simulink library "Library_Steering"  (R2023a)
settings: Solver=VariableStepAuto  StartTime=0.0  StopTime=10.0  RelTol=1e-3
undefined symbols (not defined in the file or in its folder): SteeringLeft, SteeringRight
libraries: mbd_s32k1xx_ec_toolbox x17, simulink x8, $bdroot x3
(part 1 of 2)
settings Model: Creator=cbeal  LastModifiedBy=cbeal
settings SolverCC: AlgebraicLoopSolver=TrustRegion
settings DebuggingCC: UnconnectedInputMsg=warning  UnconnectedOutputMsg=warning  UnconnectedLineMsg=warning
settings ModelReferenceCC: EnableRefExpFcnMdlSchedulingChecks=on
settings RTWCC: DLArmComputeVersion=19.05

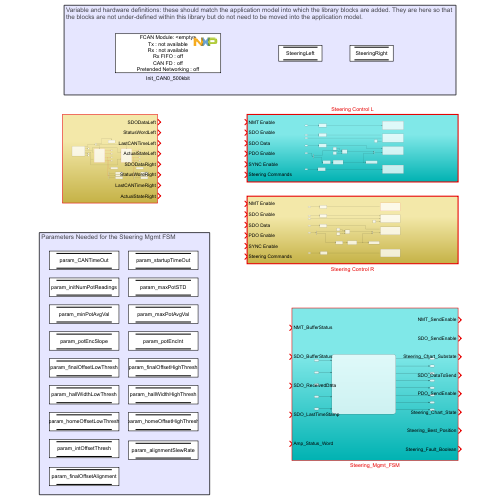
[thumbnail: Simulink's stored preview of the top-level diagram]
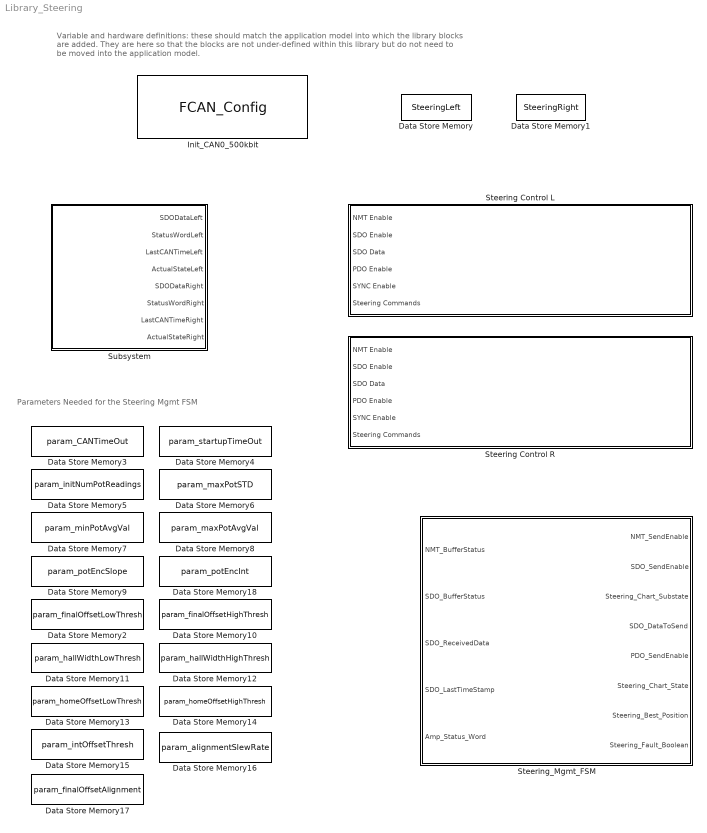
== system Library_Steering ==
  note: Parameters Needed for the Steering Mgmt FSM
  note: Variable and hardware definitions: these should match the application model into which the library blocks are added. They are here so that
      | the blocks are not under-defined within this library but do not need to be moved into the application model.
  Data Store Memory : DataStoreMemory  DataStoreName=SteeringLeft  ReadBeforeWriteMsg=warning  WriteAfterWriteMsg=warning  WriteAfterReadMsg=warning  InitialValue=zeros(15,1)  ShowAdditionalParam=off  OutDataTypeStr=uint8
  Data Store Memory1 : DataStoreMemory  DataStoreName=SteeringRight  ReadBeforeWriteMsg=warning  WriteAfterWriteMsg=warning  WriteAfterReadMsg=warning  InitialValue=zeros(15,1)  ShowAdditionalParam=off  OutDataTypeStr=uint8
  Data Store Memory10 : DataStoreMemory  DataStoreName=param_finalOffsetHighThresh  ReadBeforeWriteMsg=warning  WriteAfterWriteMsg=warning  WriteAfterReadMsg=warning  InitialValue=p1params.steering.left.finalOffsetHighThresh  ShowAdditionalParam=off  OutDataTypeStr=double
  Data Store Memory11 : DataStoreMemory  DataStoreName=param_hallWidthLowThresh  ReadBeforeWriteMsg=warning  WriteAfterWriteMsg=warning  WriteAfterReadMsg=warning  InitialValue=p1params.steering.left.hallWidthLowThresh  ShowAdditionalParam=off  OutDataTypeStr=double
  Data Store Memory12 : DataStoreMemory  DataStoreName=param_hallWidthHighThresh  ReadBeforeWriteMsg=warning  WriteAfterWriteMsg=warning  WriteAfterReadMsg=warning  InitialValue=p1params.steering.left.hallWidthHighThresh  ShowAdditionalParam=off  OutDataTypeStr=double
  Data Store Memory13 : DataStoreMemory  DataStoreName=param_homeOffsetLowThresh  ReadBeforeWriteMsg=warning  WriteAfterWriteMsg=warning  WriteAfterReadMsg=warning  InitialValue=p1params.steering.left.homeOffsetLowThresh  ShowAdditionalParam=off  OutDataTypeStr=double
  Data Store Memory14 : DataStoreMemory  DataStoreName=param_homeOffsetHighThresh  ReadBeforeWriteMsg=warning  WriteAfterWriteMsg=warning  WriteAfterReadMsg=warning  InitialValue=p1params.steering.left.homeOffsetHighThresh  ShowAdditionalParam=off  OutDataTypeStr=double
  Data Store Memory15 : DataStoreMemory  DataStoreName=param_intOffsetThresh  ReadBeforeWriteMsg=warning  WriteAfterWriteMsg=warning  WriteAfterReadMsg=warning  InitialValue=p1params.steering.left.intOffsetThresh  ShowAdditionalParam=off  OutDataTypeStr=double
  Data Store Memory16 : DataStoreMemory  DataStoreName=param_alignmentSlewRate  ReadBeforeWriteMsg=warning  WriteAfterWriteMsg=warning  WriteAfterReadMsg=warning  InitialValue=p1params.steering.left.alignmentSlewRate  ShowAdditionalParam=off  OutDataTypeStr=double
  Data Store Memory17 : DataStoreMemory  DataStoreName=param_finalOffsetAlignment  ReadBeforeWriteMsg=warning  WriteAfterWriteMsg=warning  WriteAfterReadMsg=warning  InitialValue=p1params.steering.left.finalOffsetAlignment  ShowAdditionalParam=off  OutDataTypeStr=double
  Data Store Memory18 : DataStoreMemory  DataStoreName=param_potEncInt  ReadBeforeWriteMsg=warning  WriteAfterWriteMsg=warning  WriteAfterReadMsg=warning  InitialValue=p1params.steering.left.potEncInt  ShowAdditionalParam=off  OutDataTypeStr=double
  Data Store Memory2 : DataStoreMemory  DataStoreName=param_finalOffsetLowThresh  ReadBeforeWriteMsg=warning  WriteAfterWriteMsg=warning  WriteAfterReadMsg=warning  InitialValue=p1params.steering.left.finalOffsetLowThresh  ShowAdditionalParam=off  OutDataTypeStr=double
  Data Store Memory3 : DataStoreMemory  DataStoreName=param_CANTimeOut  ReadBeforeWriteMsg=warning  WriteAfterWriteMsg=warning  WriteAfterReadMsg=warning  ShowAdditionalParam=off  OutDataTypeStr=double
  Data Store Memory4 : DataStoreMemory  DataStoreName=param_startupTimeOut  ReadBeforeWriteMsg=warning  WriteAfterWriteMsg=warning  WriteAfterReadMsg=warning  ShowAdditionalParam=off  OutDataTypeStr=double
  Data Store Memory5 : DataStoreMemory  DataStoreName=param_initNumPotReadings  ReadBeforeWriteMsg=warning  WriteAfterWriteMsg=warning  WriteAfterReadMsg=warning  InitialValue=p1params.steering.left.initNumPotReadings  ShowAdditionalParam=off  OutDataTypeStr=double
  Data Store Memory6 : DataStoreMemory  DataStoreName=param_maxPotSTD  ReadBeforeWriteMsg=warning  WriteAfterWriteMsg=warning  WriteAfterReadMsg=warning  InitialValue=p1params.steering.left.maxPotSTD  ShowAdditionalParam=off  OutDataTypeStr=double
  Data Store Memory7 : DataStoreMemory  DataStoreName=param_minPotAvgVal  ReadBeforeWriteMsg=warning  WriteAfterWriteMsg=warning  WriteAfterReadMsg=warning  InitialValue=p1params.steering.left.minPotAvgVal  ShowAdditionalParam=off  OutDataTypeStr=double
  Data Store Memory8 : DataStoreMemory  DataStoreName=param_maxPotAvgVal  ReadBeforeWriteMsg=warning  WriteAfterWriteMsg=warning  WriteAfterReadMsg=warning  InitialValue=p1params.steering.left.maxPotAvgVal  ShowAdditionalParam=off  OutDataTypeStr=double
  Data Store Memory9 : DataStoreMemory  DataStoreName=param_potEncSlope  ReadBeforeWriteMsg=warning  WriteAfterWriteMsg=warning  WriteAfterReadMsg=warning  InitialValue=p1params.steering.left.potEncSlope  ShowAdditionalParam=off  OutDataTypeStr=double
  Init_CAN0_500kbit : mbd_s32k1xx_ec_toolbox/Communication Blocks/CAN Blocks/FCAN_Config  Priority=1  can_instance=<empty>  can_mode=Normal mode  can_max_num_mb=0  can_rx=not available  can_tx=not available  show_adv_opts=off  can_clk_src=Peripheral clock  bitrate=500  bitrate_adv_opts=off  can_presdiv=7  can_rjw=3  can_pseg1=6  can_pseg2=3  can_propseg=7  can_cbt_presdiv=9  can_cbt_rjw=0  can_cbt_pseg1=3  can_cbt_pseg2=3  can_cbt_propseg=6  can_fd_enable=off  can_payload=8  can_rxfifo_enable=off  can_fifo_id_filter_extended=off  can_fifo_id_filter_remote=off  can_num_id_filters=8  can_fifo_id_format=A  can_fifo_id_filter={'0x0', '0x0', '0x0', '0x0', '0x0', '0x0', '0x0', '0x0'}  can_pn_enable=off  can_wakeup_match=off  can_wakeup_timeout=off  can_timeout_en=off  can_match_timeout=1  can_multiple_matches_en=off  can_num_matches=1  can_idfilter_extendedid=off  can_idfilter_remoteframe=off  can_idfilter_type=Match exact  can_idfilter_id1=0  can_idfilter_id2=0  can_payloadfilter_enable=on  can_payloadfilter_dlclow=0  can_payloadfilter_dlchigh=0  can_payloadfilter_type=Match exact  can_payloadfilter_payload1_b0=0  can_payloadfilter_payload1_b1=0  can_payloadfilter_payload1_b2=0  can_payloadfilter_payload1_b3=0  can_payloadfilter_payload1_b4=0  can_payloadfilter_payload1_b5=0  can_payloadfilter_payload1_b6=0  can_payloadfilter_payload1_b7=0  can_payloadfilter_payload2_b0=0  can_payloadfilter_payload2_b1=0  can_payloadfilter_payload2_b2=0  can_payloadfilter_payload2_b3=0  can_payloadfilter_payload2_b4=0  can_payloadfilter_payload2_b5=0  can_payloadfilter_payload2_b6=0  can_payloadfilter_payload2_b7=0
  Steering Control L : Subsystem  TreatAsAtomicUnit=on
      settings: RTWSystemCode=Nonreusable function
  Steering Control R : Subsystem  TreatAsAtomicUnit=on
      settings: RTWSystemCode=Nonreusable function
  Steering_Mgmt_FSM : Subsystem
  Subsystem : Subsystem

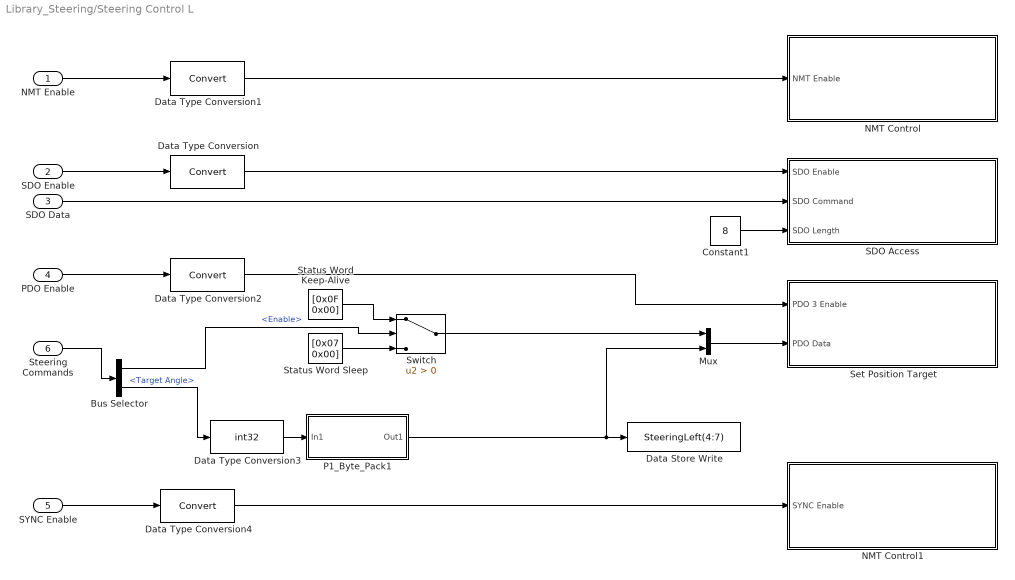
== system Library_Steering/Steering Control L ==
  NMT Enable : Inport
  SDO Enable : Inport  Port=2
  SDO Data : Inport  Port=3
  PDO Enable : Inport  Port=4
  SYNC Enable : Inport  Port=5
  Steering Commands : Inport  Port=6
  Bus Selector : BusSelector  OutputSignals=Enable,Target Angle
  Constant1 : Constant  Value=8  OutDataTypeStr=uint8
  Data Store Write : DataStoreWrite  DataStoreName=SteeringLeft  DataStoreElements=SteeringLeft(4:7)  IndexOptions=Index vector (dialog)  Indices=1  OutputSizes=1
  Data Type Conversion{,1..2,4} (4 alike) : DataTypeConversion  SaturateOnIntegerOverflow=off  RndMeth=Floor
  Data Type Conversion3 : DataTypeConversion  OutDataTypeStr=int32  SaturateOnIntegerOverflow=off  RndMeth=Floor
  Mux : Mux  Inputs=2
  NMT Control : Subsystem
  NMT Control1 : Subsystem
  P1_Byte_Pack1 : Subsystem
  SDO Access : Subsystem
  Set Position Target : Subsystem  TreatAsAtomicUnit=on
      settings: RTWSystemCode=Nonreusable function
  Status Word Keep-Alive : Constant  Value=[0x0F 0x00]  OutDataTypeStr=uint8
  Status Word Sleep : Constant  Value=[0x07 0x00]  OutDataTypeStr=uint8
  Switch : Switch  Criteria=u2 > Threshold  SaturateOnIntegerOverflow=off  InputSameDT=off
  wires:
  Switch/1 -> Mux/1
  Bus Selector/1 -> Switch/2  "<Enable>"
  Status Word Sleep/1 -> Switch/3
  Bus Selector/2 -> Data Type Conversion3/1  "<Target Angle>"
  SDO Data/1 -> SDO Access/2(SDO Command)
  NMT Enable/1 -> Data Type Conversion1/1
  SDO Enable/1 -> Data Type Conversion/1
  Status Word Keep-Alive/1 -> Switch/1
  Mux/1 -> Set Position Target/2(PDO Data)
  Constant1/1 -> SDO Access/3(SDO Length)
  Data Type Conversion2/1 -> Set Position Target/1(PDO 3 Enable)
  Data Type Conversion1/1 -> NMT Control/1(NMT Enable)
  Data Type Conversion/1 -> SDO Access/1(SDO Enable)
  PDO Enable/1 -> Data Type Conversion2/1
  P1_Byte_Pack1/1(Out1) -> Data Store Write/1, Mux/2
  Steering Commands/1 -> Bus Selector/1
  Data Type Conversion3/1 -> P1_Byte_Pack1/1(In1)
  SYNC Enable/1 -> Data Type Conversion4/1
  Data Type Conversion4/1 -> NMT Control1/1(SYNC Enable)

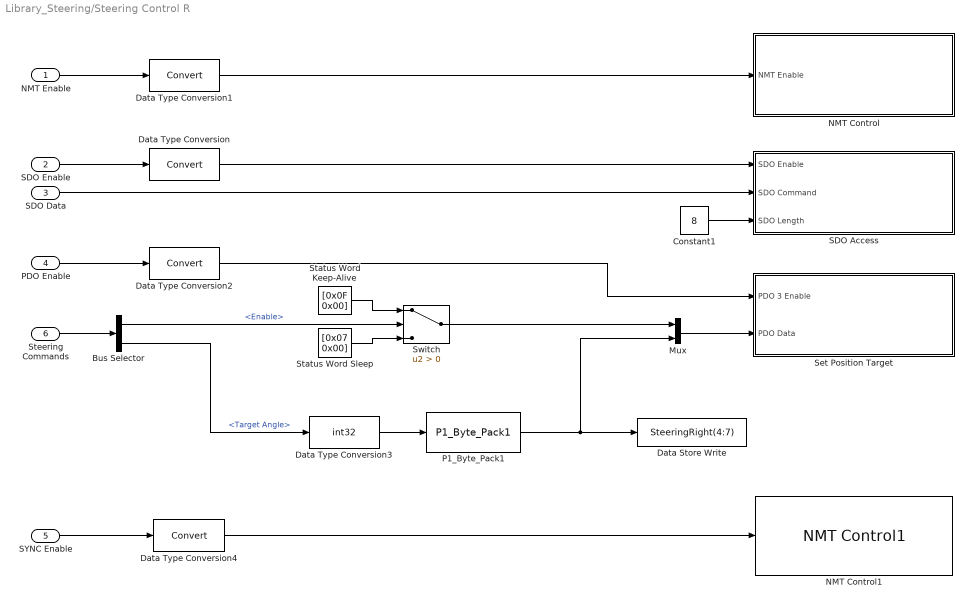
== system Library_Steering/Steering Control R ==
  NMT Enable : Inport
  SDO Enable : Inport  Port=2
  SDO Data : Inport  Port=3
  PDO Enable : Inport  Port=4
  SYNC Enable : Inport  Port=5
  Steering Commands : Inport  Port=6
  Bus Selector : BusSelector  OutputSignals=Enable,Target Angle
  Constant1 : Constant  Value=8  OutDataTypeStr=uint8
  Data Store Write : DataStoreWrite  DataStoreName=SteeringRight  DataStoreElements=SteeringRight(4:7)  IndexOptions=Index vector (dialog)  Indices=1  OutputSizes=1
  Data Type Conversion{,1..2,4} (4 alike) : DataTypeConversion  SaturateOnIntegerOverflow=off  RndMeth=Floor
  Data Type Conversion3 : DataTypeConversion  OutDataTypeStr=int32  SaturateOnIntegerOverflow=off  RndMeth=Floor
  Mux : Mux  Inputs=2
  NMT Control : Subsystem
  NMT Control1 : $bdroot/Steering Control L/NMT Control1  SystemSampleTime=-1  VariantActivationTime=update diagram  Latency=0  AutoFrameSizeCalculation=off
  P1_Byte_Pack1 : $bdroot/Steering Control L/P1_Byte_Pack1  SystemSampleTime=-1  VariantActivationTime=update diagram  Latency=0  AutoFrameSizeCalculation=off
  SDO Access : Subsystem
  Set Position Target : Subsystem  TreatAsAtomicUnit=on
      settings: RTWSystemCode=Nonreusable function
  Status Word Keep-Alive : Constant  Value=[0x0F 0x00]  OutDataTypeStr=uint8
  Status Word Sleep : Constant  Value=[0x07 0x00]  OutDataTypeStr=uint8
  Switch : Switch  Criteria=u2 > Threshold  SaturateOnIntegerOverflow=off  InputSameDT=off
  wires:
  Mux/1 -> Set Position Target/2(PDO Data)
  Switch/1 -> Mux/1
  Status Word Sleep/1 -> Switch/3
  Status Word Keep-Alive/1 -> Switch/1
  Bus Selector/1 -> Switch/2  "<Enable>"
  SDO Data/1 -> SDO Access/2(SDO Command)
  NMT Enable/1 -> Data Type Conversion1/1
  SDO Enable/1 -> Data Type Conversion/1
  Constant1/1 -> SDO Access/3(SDO Length)
  Data Type Conversion2/1 -> Set Position Target/1(PDO 3 Enable)
  Data Type Conversion1/1 -> NMT Control/1(NMT Enable)
  Data Type Conversion/1 -> SDO Access/1(SDO Enable)
  PDO Enable/1 -> Data Type Conversion2/1
  Steering Commands/1 -> Bus Selector/1
  Data Type Conversion3/1 -> P1_Byte_Pack1/1
  P1_Byte_Pack1/1 -> Data Store Write/1, Mux/2
  Bus Selector/2 -> Data Type Conversion3/1  "<Target Angle>"
  SYNC Enable/1 -> Data Type Conversion4/1
  Data Type Conversion4/1 -> NMT Control1/1

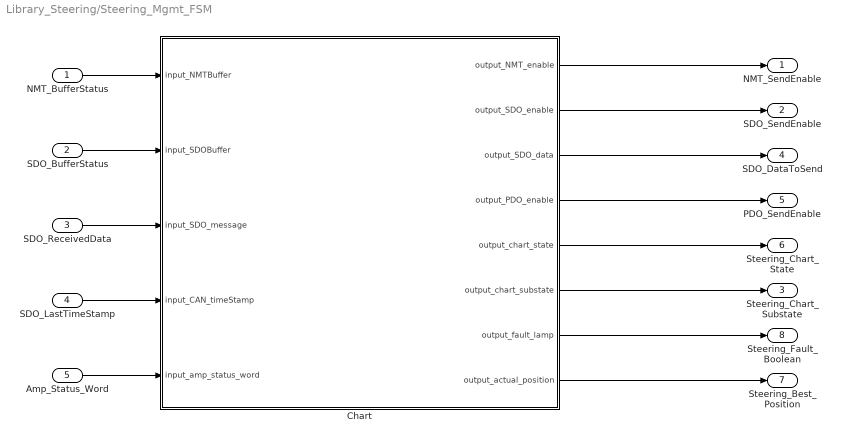
== system Library_Steering/Steering_Mgmt_FSM ==
  NMT_BufferStatus : Inport
  SDO_BufferStatus : Inport  Port=2
  SDO_ReceivedData : Inport  Port=3
  SDO_LastTimeStamp : Inport  Port=4
  Amp_Status_Word : Inport  Port=5
  Chart : Stateflow chart  TreatAsAtomicUnit=on
      settings: RTWSystemCode=Nonreusable function
  NMT_SendEnable : Outport
  SDO_SendEnable : Outport  Port=2
  Steering_Chart_Substate : Outport  Port=3
  SDO_DataToSend : Outport  Port=4
  PDO_SendEnable : Outport  Port=5
  Steering_Chart_State : Outport  Port=6
  Steering_Best_Position : Outport  Port=7
  Steering_Fault_Boolean : Outport  Port=8
  wires:
  NMT_BufferStatus/1 -> Chart/1(input_NMTBuffer)
  SDO_BufferStatus/1 -> Chart/2(input_SDOBuffer)
  SDO_LastTimeStamp/1 -> Chart/4(input_CAN_timeStamp)
  SDO_ReceivedData/1 -> Chart/3(input_SDO_message)
  Chart/1(output_NMT_enable) -> NMT_SendEnable/1
  Chart/6(output_chart_substate) -> Steering_Chart_Substate/1
  Chart/2(output_SDO_enable) -> SDO_SendEnable/1
  Chart/3(output_SDO_data) -> SDO_DataToSend/1
  Chart/4(output_PDO_enable) -> PDO_SendEnable/1
  Chart/5(output_chart_state) -> Steering_Chart_State/1
  Chart/7(output_fault_lamp) -> Steering_Fault_Boolean/1
  Chart/8(output_actual_position) -> Steering_Best_Position/1
  Amp_Status_Word/1 -> Chart/5(input_amp_status_word)

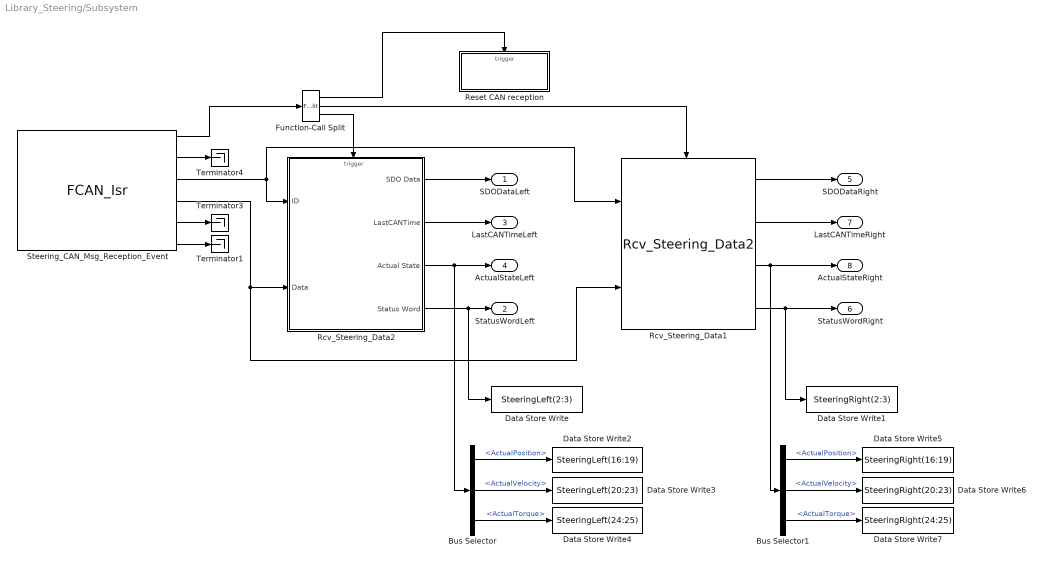
== system Library_Steering/Subsystem ==
  Bus Selector : BusSelector  OutputSignals=ActualPosition,ActualVelocity,ActualTorque
  Bus Selector1 : BusSelector  OutputSignals=ActualPosition,ActualVelocity,ActualTorque
  Data Store Write : DataStoreWrite  DataStoreName=SteeringLeft  DataStoreElements=SteeringLeft(2:3)  IndexOptions=Index vector (dialog)  Indices=1  OutputSizes=1
  Data Store Write1 : DataStoreWrite  DataStoreName=SteeringRight  DataStoreElements=SteeringRight(2:3)  IndexOptions=Index vector (dialog)  Indices=1  OutputSizes=1
  Data Store Write2 : DataStoreWrite  DataStoreName=SteeringLeft  DataStoreElements=SteeringLeft(16:19)  IndexOptions=Index vector (dialog)  Indices=1  OutputSizes=1
  Data Store Write3 : DataStoreWrite  DataStoreName=SteeringLeft  DataStoreElements=SteeringLeft(20:23)  IndexOptions=Index vector (dialog)  Indices=1  OutputSizes=1
  Data Store Write4 : DataStoreWrite  DataStoreName=SteeringLeft  DataStoreElements=SteeringLeft(24:25)  IndexOptions=Index vector (dialog)  Indices=1  OutputSizes=1
  Data Store Write5 : DataStoreWrite  DataStoreName=SteeringRight  DataStoreElements=SteeringRight(16:19)  IndexOptions=Index vector (dialog)  Indices=1  OutputSizes=1
  Data Store Write6 : DataStoreWrite  DataStoreName=SteeringRight  DataStoreElements=SteeringRight(20:23)  IndexOptions=Index vector (dialog)  Indices=1  OutputSizes=1
  Data Store Write7 : DataStoreWrite  DataStoreName=SteeringRight  DataStoreElements=SteeringRight(24:25)  IndexOptions=Index vector (dialog)  Indices=1  OutputSizes=1
  Function-Call Split : FunctionCallSplit  IconShape=distinctive  NumOutputPorts=3  OutputPortLayout=default
  Rcv_Steering_Data1 : $bdroot/Subsystem/Rcv_Steering_Data2  ampAddress=hex2dec('D')
  Rcv_Steering_Data2 : Subsystem  TreatAsAtomicUnit=on  mask{ampAddress=hex2dec('B')}
      mask prompts: ampAddress "Amplifier ID (Enter as: hex2dec('N'))"
      settings: RTWSystemCode=Nonreusable function
  Reset CAN reception : Subsystem  TreatAsAtomicUnit=on
  Steering_CAN_Msg_Reception_Event : mbd_s32k1xx_ec_toolbox/Communication Blocks/CAN Blocks/FCAN_Isr  Priority=2  can_instance=0  can_event=Rx Complete
  Terminator1 : Terminator
  Terminator3 : Terminator
  Terminator4 : Terminator
  SDODataLeft : Outport
  StatusWordLeft : Outport  Port=2
  LastCANTimeLeft : Outport  Port=3
  ActualStateLeft : Outport  Port=4
  SDODataRight : Outport  Port=5
  StatusWordRight : Outport  Port=6
  LastCANTimeRight : Outport  Port=7
  ActualStateRight : Outport  Port=8
  wires:
  Function-Call Split/1 -> Reset CAN reception/Trigger
  Steering_CAN_Msg_Reception_Event/5 -> Terminator3/1
  Steering_CAN_Msg_Reception_Event/2 -> Terminator4/1
  Steering_CAN_Msg_Reception_Event/1 -> Function-Call Split/1
  Steering_CAN_Msg_Reception_Event/3 -> Rcv_Steering_Data1/1, Rcv_Steering_Data2/1(ID)
  Rcv_Steering_Data2/1(SDO Data) -> SDODataLeft/1
  Rcv_Steering_Data2/2(LastCANTime) -> LastCANTimeLeft/1
  Rcv_Steering_Data2/3(Actual State) -> Bus Selector/1, ActualStateLeft/1
  Steering_CAN_Msg_Reception_Event/6 -> Terminator1/1
  Steering_CAN_Msg_Reception_Event/4 -> Rcv_Steering_Data1/2, Rcv_Steering_Data2/2(Data)
  Function-Call Split/3 -> Rcv_Steering_Data2/Trigger
  Function-Call Split/2 -> Rcv_Steering_Data1/Trigger
  Rcv_Steering_Data2/4(Status Word) -> Data Store Write/1, StatusWordLeft/1
  Rcv_Steering_Data1/1 -> SDODataRight/1
  Rcv_Steering_Data1/2 -> LastCANTimeRight/1
  Rcv_Steering_Data1/3 -> Bus Selector1/1, ActualStateRight/1
  Rcv_Steering_Data1/4 -> Data Store Write1/1, StatusWordRight/1
  Bus Selector/1 -> Data Store Write2/1  "<ActualPosition>"
  Bus Selector/2 -> Data Store Write3/1  "<ActualVelocity>"
  Bus Selector/3 -> Data Store Write4/1  "<ActualTorque>"
  Bus Selector1/3 -> Data Store Write7/1  "<ActualTorque>"
  Bus Selector1/2 -> Data Store Write6/1  "<ActualVelocity>"
  Bus Selector1/1 -> Data Store Write5/1  "<ActualPosition>"

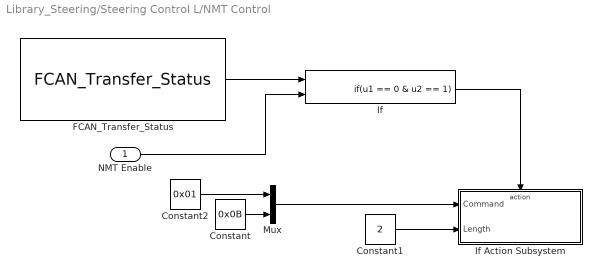
== system Library_Steering/Steering Control L/NMT Control ==
  NMT Enable : Inport
  Constant : Constant  Value=0x0B  OutDataTypeStr=uint8
  Constant1 : Constant  Value=2  OutDataTypeStr=uint8
  Constant2 : Constant  Value=0x01  OutDataTypeStr=uint8
  FCAN_Transfer_Status : mbd_s32k1xx_ec_toolbox/Communication Blocks/CAN Blocks/FCAN_Transfer_Status  can_instance=0  can_mb_idx=1
  If : If  NumInputs=2  IfExpression=u1 == 0 & u2 == 1  ShowElse=off
  If Action Subsystem : Subsystem  TreatAsAtomicUnit=on
      settings: RTWSystemCode=Nonreusable function
  Mux : Mux  Inputs=2
  wires:
  Constant1/1 -> If Action Subsystem/2(Length)
  NMT Enable/1 -> If/2
  FCAN_Transfer_Status/1 -> If/1
  If/1 -> If Action Subsystem/Action
  Mux/1 -> If Action Subsystem/1(Command)
  Constant2/1 -> Mux/1
  Constant/1 -> Mux/2

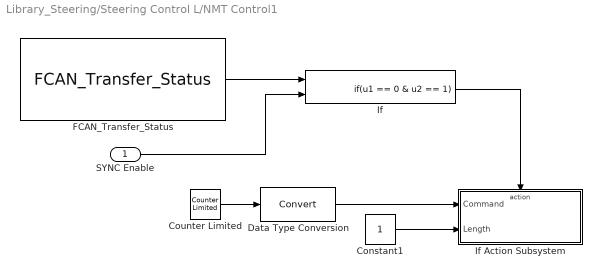
== system Library_Steering/Steering Control L/NMT Control1 ==
  SYNC Enable : Inport
  Constant1 : Constant  OutDataTypeStr=uint8
  Counter Limited : simulink/Sources/Counter Limited  uplimit=255  tsamp=-1
  Data Type Conversion : DataTypeConversion  SaturateOnIntegerOverflow=off  RndMeth=Floor
  FCAN_Transfer_Status : mbd_s32k1xx_ec_toolbox/Communication Blocks/CAN Blocks/FCAN_Transfer_Status  can_instance=0  can_mb_idx=1
  If : If  NumInputs=2  IfExpression=u1 == 0 & u2 == 1  ShowElse=off
  If Action Subsystem : Subsystem  TreatAsAtomicUnit=on
      settings: RTWSystemCode=Nonreusable function
  wires:
  If/1 -> If Action Subsystem/Action
  FCAN_Transfer_Status/1 -> If/1
  SYNC Enable/1 -> If/2
  Constant1/1 -> If Action Subsystem/2(Length)
  Counter Limited/1 -> Data Type Conversion/1
  Data Type Conversion/1 -> If Action Subsystem/1(Command)

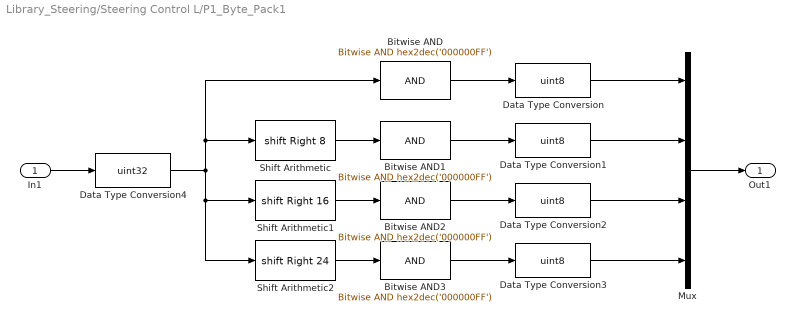
== system Library_Steering/Steering Control L/P1_Byte_Pack1 ==
  In1 : Inport
  Bitwise AND{,1..3} (4 alike) : simulink/Logic and Bit Operations/Bitwise Operator  logicop=AND  UseBitMask=on  BitMask=hex2dec('000000FF')  BitMaskRealWorld=Stored Integer
  Data Type Conversion{,1..3} (4 alike) : DataTypeConversion  OutDataTypeStr=uint8  ConvertRealWorld=Stored Integer (SI)  SaturateOnIntegerOverflow=off  RndMeth=Floor
  Data Type Conversion4 : DataTypeConversion  OutDataTypeStr=uint32  ConvertRealWorld=Stored Integer (SI)  SaturateOnIntegerOverflow=off  RndMeth=Floor
  Mux : Mux
  Shift Arithmetic : ArithShift  BitShiftNumber=8  BitShiftDirection=Right
  Shift Arithmetic1 : ArithShift  BitShiftNumber=16  BitShiftDirection=Right
  Shift Arithmetic2 : ArithShift  BitShiftNumber=24  BitShiftDirection=Right
  Out1 : Outport
  wires:
  Data Type Conversion3/1 -> Mux/4
  Data Type Conversion2/1 -> Mux/3
  Data Type Conversion1/1 -> Mux/2
  Data Type Conversion/1 -> Mux/1
  Data Type Conversion4/1 -> Shift Arithmetic2/1, Shift Arithmetic1/1, Shift Arithmetic/1, Bitwise AND/1
  Bitwise AND/1 -> Data Type Conversion/1
  Shift Arithmetic/1 -> Bitwise AND1/1
  Mux/1 -> Out1/1
  In1/1 -> Data Type Conversion4/1
  Bitwise AND1/1 -> Data Type Conversion1/1
  Bitwise AND2/1 -> Data Type Conversion2/1
  Bitwise AND3/1 -> Data Type Conversion3/1
  Shift Arithmetic1/1 -> Bitwise AND2/1
  Shift Arithmetic2/1 -> Bitwise AND3/1

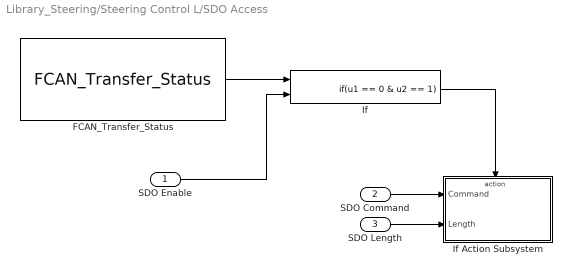
== system Library_Steering/Steering Control L/SDO Access ==
  SDO Enable : Inport
  SDO Command : Inport  Port=2
  SDO Length : Inport  Port=3
  FCAN_Transfer_Status : mbd_s32k1xx_ec_toolbox/Communication Blocks/CAN Blocks/FCAN_Transfer_Status  can_instance=0  can_mb_idx=3
  If : If  NumInputs=2  IfExpression=u1 == 0 & u2 == 1  ShowElse=off
  If Action Subsystem : Subsystem  TreatAsAtomicUnit=on
      settings: RTWSystemCode=Nonreusable function
  wires:
  If/1 -> If Action Subsystem/Action
  FCAN_Transfer_Status/1 -> If/1
  SDO Enable/1 -> If/2
  SDO Command/1 -> If Action Subsystem/1(Command)
  SDO Length/1 -> If Action Subsystem/2(Length)

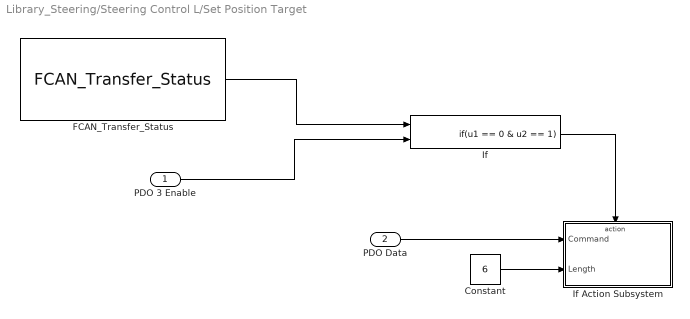
== system Library_Steering/Steering Control L/Set Position Target ==
  PDO 3 Enable : Inport
  PDO Data : Inport  Port=2
  Constant : Constant  Value=6  OutDataTypeStr=uint8
  FCAN_Transfer_Status : mbd_s32k1xx_ec_toolbox/Communication Blocks/CAN Blocks/FCAN_Transfer_Status  can_instance=0  can_mb_idx=5
  If : If  NumInputs=2  IfExpression=u1 == 0 & u2 == 1  ShowElse=off
  If Action Subsystem : Subsystem  TreatAsAtomicUnit=on
      settings: RTWSystemCode=Nonreusable function
  wires:
  FCAN_Transfer_Status/1 -> If/1
  PDO 3 Enable/1 -> If/2
  PDO Data/1 -> If Action Subsystem/1(Command)
  Constant/1 -> If Action Subsystem/2(Length)
  If/1 -> If Action Subsystem/Action

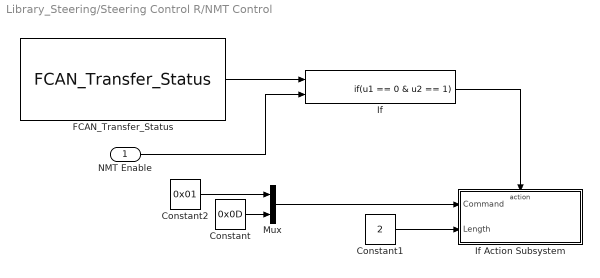
== system Library_Steering/Steering Control R/NMT Control ==
  NMT Enable : Inport
  Constant : Constant  Value=0x0D  OutDataTypeStr=uint8
  Constant1 : Constant  Value=2  OutDataTypeStr=uint8
  Constant2 : Constant  Value=0x01  OutDataTypeStr=uint8
  FCAN_Transfer_Status : mbd_s32k1xx_ec_toolbox/Communication Blocks/CAN Blocks/FCAN_Transfer_Status  can_instance=0  can_mb_idx=7
  If : If  NumInputs=2  IfExpression=u1 == 0 & u2 == 1  ShowElse=off
  If Action Subsystem : Subsystem  TreatAsAtomicUnit=on
      settings: RTWSystemCode=Nonreusable function
  Mux : Mux  Inputs=2
  wires:
  Constant1/1 -> If Action Subsystem/2(Length)
  NMT Enable/1 -> If/2
  FCAN_Transfer_Status/1 -> If/1
  If/1 -> If Action Subsystem/Action
  Mux/1 -> If Action Subsystem/1(Command)
  Constant2/1 -> Mux/1
  Constant/1 -> Mux/2

== system Library_Steering/Steering Control R/SDO Access ==
  SDO Enable : Inport
  SDO Command : Inport  Port=2
  SDO Length : Inport  Port=3
  FCAN_Transfer_Status : mbd_s32k1xx_ec_toolbox/Communication Blocks/CAN Blocks/FCAN_Transfer_Status  can_instance=0  can_mb_idx=9
  If : If  NumInputs=2  IfExpression=u1 == 0 & u2 == 1  ShowElse=off
  If Action Subsystem : Subsystem  TreatAsAtomicUnit=on
      settings: RTWSystemCode=Nonreusable function
  wires:
  If/1 -> If Action Subsystem/Action
  FCAN_Transfer_Status/1 -> If/1
  SDO Enable/1 -> If/2
  SDO Command/1 -> If Action Subsystem/1(Command)
  SDO Length/1 -> If Action Subsystem/2(Length)

== system Library_Steering/Steering Control R/Set Position Target ==
  PDO 3 Enable : Inport
  PDO Data : Inport  Port=2
  Constant : Constant  Value=6  OutDataTypeStr=uint8
  FCAN_Transfer_Status : mbd_s32k1xx_ec_toolbox/Communication Blocks/CAN Blocks/FCAN_Transfer_Status  can_instance=0  can_mb_idx=11
  If : If  NumInputs=2  IfExpression=u1 == 0 & u2 == 1  ShowElse=off
  If Action Subsystem : Subsystem  TreatAsAtomicUnit=on
      settings: RTWSystemCode=Nonreusable function
  wires:
  FCAN_Transfer_Status/1 -> If/1
  PDO 3 Enable/1 -> If/2
  PDO Data/1 -> If Action Subsystem/1(Command)
  Constant/1 -> If Action Subsystem/2(Length)
  If/1 -> If Action Subsystem/Action

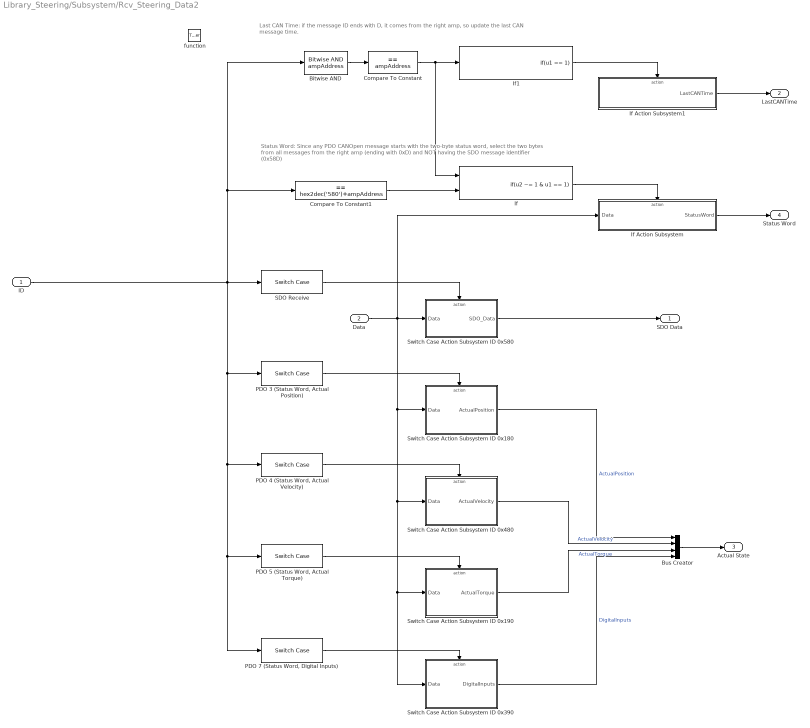
== system Library_Steering/Subsystem/Rcv_Steering_Data2 ==
  note: Status Word: Since any PDO CANOpen message starts with the two-byte status word, select the two bytes from all messages from the right amp (ending with 0xD) and NOT
      | having the SDO message identifier (0x58D)
  note: Last CAN Time: if the message ID ends with D, it comes from the right amp, so update the last CAN message time.
  ID : Inport
  Data : Inport  Port=2
  function : TriggerPort  TriggerType=function-call  VariantControl=Variant
  Bitwise AND : simulink/Logic and Bit Operations/Bitwise Operator  logicop=AND  UseBitMask=on  BitMask=ampAddress  BitMaskRealWorld=Stored Integer
  Bus Creator : BusCreator  Inputs=4
  Compare To Constant : simulink/Logic and Bit Operations/Compare To Constant  relop===  const=ampAddress  OutDataTypeStr=boolean
  Compare To Constant1 : simulink/Logic and Bit Operations/Compare To Constant  relop===  const=hex2dec('580')+ampAddress  OutDataTypeStr=boolean
  If : If  NumInputs=2  IfExpression=u2 ~= 1 & u1 == 1  ShowElse=off
  If Action Subsystem : Subsystem  TreatAsAtomicUnit=on
      settings: RTWSystemCode=Nonreusable function
  If Action Subsystem1 : Subsystem  TreatAsAtomicUnit=on
      settings: RTWSystemCode=Nonreusable function
  If1 : If  IfExpression=u1 == 1  ShowElse=off
  "PDO 3 (Status Word, Actual Position)" : SwitchCase  CaseConditions={hex2dec('380')+ampAddress}  ShowDefaultCase=off
  "PDO 4 (Status Word, Actual Velocity)" : SwitchCase  CaseConditions={hex2dec('480')+ampAddress}  ShowDefaultCase=off
  "PDO 5 (Status Word, Actual Torque)" : SwitchCase  CaseConditions={hex2dec('190')+ampAddress}  ShowDefaultCase=off
  "PDO 7 (Status Word, Digital Inputs)" : SwitchCase  CaseConditions={hex2dec('390')+ampAddress}  ShowDefaultCase=off
  SDO Receive : SwitchCase  CaseConditions={hex2dec('580')+ampAddress}  ShowDefaultCase=off
  Switch Case Action Subsystem ID 0x180 : Subsystem  TreatAsAtomicUnit=on
  Switch Case Action Subsystem ID 0x190 : Subsystem  TreatAsAtomicUnit=on
  Switch Case Action Subsystem ID 0x390 : Subsystem  TreatAsAtomicUnit=on
  Switch Case Action Subsystem ID 0x480 : Subsystem  TreatAsAtomicUnit=on
  Switch Case Action Subsystem ID 0x580 : Subsystem  TreatAsAtomicUnit=on
  SDO Data : Outport
  LastCANTime : Outport  Port=2
  Actual State : Outport  Port=3
  Status Word : Outport  Port=4
  wires:
  Compare To Constant1/1 -> If/2
  Switch Case Action Subsystem ID 0x390/1(DigitalInputs) -> Bus Creator/4  "DigitalInputs"
  Switch Case Action Subsystem ID 0x190/1(ActualTorque) -> Bus Creator/3  "ActualTorque"
  Switch Case Action Subsystem ID 0x480/1(ActualVelocity) -> Bus Creator/2  "ActualVelocity"
  Switch Case Action Subsystem ID 0x180/1(ActualPosition) -> Bus Creator/1  "ActualPosition"
  Bus Creator/1 -> Actual State/1
  "PDO 5 (Status Word, Actual Torque)"/1 -> Switch Case Action Subsystem ID 0x190/Action
  "PDO 7 (Status Word, Digital Inputs)"/1 -> Switch Case Action Subsystem ID 0x390/Action
  "PDO 4 (Status Word, Actual Velocity)"/1 -> Switch Case Action Subsystem ID 0x480/Action
  "PDO 3 (Status Word, Actual Position)"/1 -> Switch Case Action Subsystem ID 0x180/Action
  If Action Subsystem1/1(LastCANTime) -> LastCANTime/1
  ID/1 -> Bitwise AND/1, Compare To Constant1/1, SDO Receive/1, "PDO 4 (Status Word, Actual Velocity)"/1, "PDO 7 (Status Word, Digital Inputs)"/1, "PDO 5 (Status Word, Actual Torque)"/1, "PDO 3 (Status Word, Actual Position)"/1
  Switch Case Action Subsystem ID 0x580/1(SDO_Data) -> SDO Data/1
  Data/1 -> If Action Subsystem/1(Data), Switch Case Action Subsystem ID 0x580/1(Data), Switch Case Action Subsystem ID 0x390/1(Data), Switch Case Action Subsystem ID 0x190/1(Data), Switch Case Action Subsystem ID 0x480/1(Data), Switch Case Action Subsystem ID 0x180/1(Data)
  SDO Receive/1 -> Switch Case Action Subsystem ID 0x580/Action
  If/1 -> If Action Subsystem/Action
  Bitwise AND/1 -> Compare To Constant/1
  Compare To Constant/1 -> If/1, If1/1
  If Action Subsystem/1(StatusWord) -> Status Word/1
  If1/1 -> If Action Subsystem1/Action

== system Library_Steering/Subsystem/Reset CAN reception ==
  function : TriggerPort  TriggerType=function-call  VariantControl=Variant
  FCAN_Receive : mbd_s32k1xx_ec_toolbox/Communication Blocks/CAN Blocks/FCAN_Receive  can_instance=0  can_mode=Non-blocking  can_timeout_ms=0  can_mb_idx=<empty>  can_extended_id=off  can_is_remote=off  can_id=0  can_msg_mask=0  show_adv_opts=off  can_use_rxfifo=off  can_fd_enable=off

== system Library_Steering/Steering Control L/NMT Control/If Action Subsystem ==
  Command : Inport
  Length : Inport  Port=2
  Action Port : ActionPort
  Left_Amp_NMT_Access : mbd_s32k1xx_ec_toolbox/Communication Blocks/CAN Blocks/FCAN_Send  can_instance=0  can_mode=Non-blocking  can_timeout_ms=0  can_mb_idx=1  can_extended_id=off  can_is_remote=off  can_id=0  show_adv_opts=off  can_fd_enable=off  can_enable_brs=off  can_fd_padding=0
  wires:
  Length/1 -> Left_Amp_NMT_Access/2
  Command/1 -> Left_Amp_NMT_Access/1

== system Library_Steering/Steering Control L/NMT Control1/If Action Subsystem ==
  Command : Inport
  Length : Inport  Port=2
  Action Port : ActionPort
  Left_Amp_NMT_Access : mbd_s32k1xx_ec_toolbox/Communication Blocks/CAN Blocks/FCAN_Send  can_instance=0  can_mode=Non-blocking  can_timeout_ms=0  can_mb_idx=1  can_extended_id=off  can_is_remote=off  can_id=80  show_adv_opts=off  can_fd_enable=off  can_enable_brs=off  can_fd_padding=0
  wires:
  Command/1 -> Left_Amp_NMT_Access/1
  Length/1 -> Left_Amp_NMT_Access/2

== system Library_Steering/Steering Control L/SDO Access/If Action Subsystem ==
  Command : Inport
  Length : Inport  Port=2
  Action Port : ActionPort
  Left_Amp_SDO_Access : mbd_s32k1xx_ec_toolbox/Communication Blocks/CAN Blocks/FCAN_Send  can_instance=0  can_mode=Non-blocking  can_timeout_ms=0  can_mb_idx=3  can_extended_id=off  can_is_remote=off  can_id=60B  show_adv_opts=off  can_fd_enable=off  can_enable_brs=off  can_fd_padding=0
  wires:
  Length/1 -> Left_Amp_SDO_Access/2
  Command/1 -> Left_Amp_SDO_Access/1

== system Library_Steering/Steering Control L/Set Position Target/If Action Subsystem ==
  Command : Inport
  Length : Inport  Port=2
  Action Port : ActionPort
  Left_Amp_SDO_Access : mbd_s32k1xx_ec_toolbox/Communication Blocks/CAN Blocks/FCAN_Send  can_instance=0  can_mode=Non-blocking  can_timeout_ms=0  can_mb_idx=5  can_extended_id=off  can_is_remote=off  can_id=40B  show_adv_opts=off  can_fd_enable=off  can_enable_brs=off  can_fd_padding=0
  wires:
  Length/1 -> Left_Amp_SDO_Access/2
  Command/1 -> Left_Amp_SDO_Access/1

== system Library_Steering/Steering Control R/NMT Control/If Action Subsystem ==
  Command : Inport
  Length : Inport  Port=2
  Action Port : ActionPort
  Left_Amp_NMT_Access : mbd_s32k1xx_ec_toolbox/Communication Blocks/CAN Blocks/FCAN_Send  can_instance=0  can_mode=Non-blocking  can_timeout_ms=0  can_mb_idx=7  can_extended_id=off  can_is_remote=off  can_id=0  show_adv_opts=off  can_fd_enable=off  can_enable_brs=off  can_fd_padding=0
  wires:
  Length/1 -> Left_Amp_NMT_Access/2
  Command/1 -> Left_Amp_NMT_Access/1

== system Library_Steering/Steering Control R/SDO Access/If Action Subsystem ==
  Command : Inport
  Length : Inport  Port=2
  Action Port : ActionPort
  Left_Amp_SDO_Access : mbd_s32k1xx_ec_toolbox/Communication Blocks/CAN Blocks/FCAN_Send  can_instance=0  can_mode=Non-blocking  can_timeout_ms=0  can_mb_idx=9  can_extended_id=off  can_is_remote=off  can_id=60D  show_adv_opts=off  can_fd_enable=off  can_enable_brs=off  can_fd_padding=0
  wires:
  Length/1 -> Left_Amp_SDO_Access/2
  Command/1 -> Left_Amp_SDO_Access/1

== system Library_Steering/Steering Control R/Set Position Target/If Action Subsystem ==
  Command : Inport
  Length : Inport  Port=2
  Action Port : ActionPort
  Left_Amp_SDO_Access : mbd_s32k1xx_ec_toolbox/Communication Blocks/CAN Blocks/FCAN_Send  can_instance=0  can_mode=Non-blocking  can_timeout_ms=0  can_mb_idx=11  can_extended_id=off  can_is_remote=off  can_id=40D  show_adv_opts=off  can_fd_enable=off  can_enable_brs=off  can_fd_padding=0
  wires:
  Length/1 -> Left_Amp_SDO_Access/2
  Command/1 -> Left_Amp_SDO_Access/1

== system Library_Steering/Subsystem/Rcv_Steering_Data2/If Action Subsystem ==
  Data : Inport
  Action Port : ActionPort
  IC : InitialCondition  Value=uint8([hex2dec('33') 0])
  Selector : Selector  InputPortWidth=8  IndexOptions=Index vector (dialog)  Indices=[1 2]  OutputSizes=1
  StatusWord : Outport
  wires:
  Data/1 -> Selector/1
  Selector/1 -> IC/1
  IC/1 -> StatusWord/1

== system Library_Steering/Subsystem/Rcv_Steering_Data2/If Action Subsystem1 ==
  Action Port : ActionPort
  Digital Clock : DigitalClock  SampleTime=-1
  LastCANTime : Outport
  wires:
  Digital Clock/1 -> LastCANTime/1

== system Library_Steering/Subsystem/Rcv_Steering_Data2/Switch Case Action Subsystem ID 0x180 ==
  Data : Inport
  Action Port : ActionPort
  Selector1 : Selector  InputPortWidth=8  IndexOptions=Index vector (dialog)  Indices=[3:6]  OutputSizes=1
  ActualPosition : Outport
  wires:
  Selector1/1 -> ActualPosition/1
  Data/1 -> Selector1/1

== system Library_Steering/Subsystem/Rcv_Steering_Data2/Switch Case Action Subsystem ID 0x190 ==
  Data : Inport
  Action Port : ActionPort
  Selector1 : Selector  InputPortWidth=8  IndexOptions=Index vector (dialog)  Indices=[3:4]  OutputSizes=1
  ActualTorque : Outport
  wires:
  Selector1/1 -> ActualTorque/1
  Data/1 -> Selector1/1

== system Library_Steering/Subsystem/Rcv_Steering_Data2/Switch Case Action Subsystem ID 0x390 ==
  Data : Inport
  Action Port : ActionPort
  Selector1 : Selector  InputPortWidth=8  IndexOptions=Index vector (dialog)  Indices=[3:6]  OutputSizes=1
  DigitalInputs : Outport
  wires:
  Selector1/1 -> DigitalInputs/1
  Data/1 -> Selector1/1

== system Library_Steering/Subsystem/Rcv_Steering_Data2/Switch Case Action Subsystem ID 0x480 ==
  Data : Inport
  Action Port : ActionPort
  Selector1 : Selector  InputPortWidth=8  IndexOptions=Index vector (dialog)  Indices=[3:6]  OutputSizes=1
  ActualVelocity : Outport
  wires:
  Data/1 -> Selector1/1
  Selector1/1 -> ActualVelocity/1

== system Library_Steering/Subsystem/Rcv_Steering_Data2/Switch Case Action Subsystem ID 0x580 ==
  Data : Inport
  Action Port : ActionPort
  SDO_Data : Outport
  wires:
  Data/1 -> SDO_Data/1
